simulink model "CDMA_RX_TX_with_UWA_pathloss_channel"  (Simulink 7.7)
settings: Solver=ode45  StartTime=0.0  StopTime=1  RelTol=1e-3
settings Model: Creator=iPRATEEK  LastModifiedBy=iPRATEEK

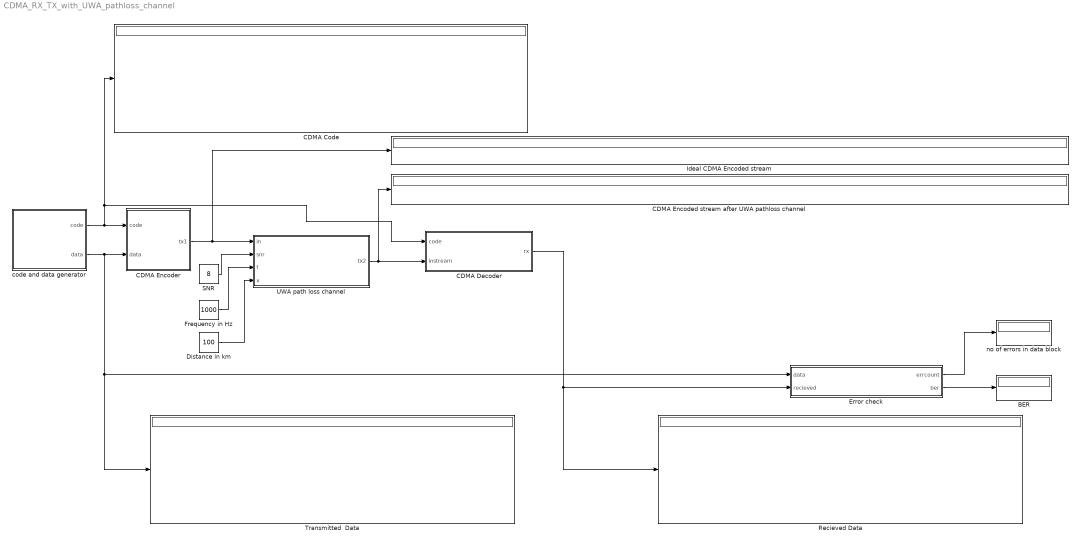
== system CDMA_RX_TX_with_UWA_pathloss_channel ==
  "BER " : Display
      settings: Format=short_e
  CDMA Code : Display
  CDMA Decoder : Stateflow chart  TreatAsAtomicUnit=on
  CDMA Encoded stream after UWA pathloss channel : Display
  CDMA Encoder : Stateflow chart  TreatAsAtomicUnit=on
  Distance in km : Constant  Value=100
  Error check : Stateflow chart  TreatAsAtomicUnit=on
  Frequency in Hz : Constant  Value=1000
  Ideal CDMA Encoded stream : Display
  Recieved Data : Display
  SNR : Constant  Value=8
  "Transmitted  Data " : Display
  UWA path loss channel : Stateflow chart  TreatAsAtomicUnit=on
  code and data generator : Stateflow chart  TreatAsAtomicUnit=on
  no of errors in data block : Display
  wires:
  code and data generator/1(code) -> CDMA Encoder/1(code), CDMA Decoder/1(code), CDMA Code/1
  code and data generator/2(data) -> CDMA Encoder/2(data), "Transmitted  Data "/1, Error check/1(data)
  CDMA Encoder/1(tx1) -> UWA path loss channel/1(in), Ideal CDMA Encoded stream/1
  SNR/1 -> UWA path loss channel/2(snr)
  CDMA Decoder/1(rx) -> Recieved Data/1, Error check/2(recieved)
  Error check/1(errcount) -> no of errors in data block/1
  Error check/2(ber) -> "BER "/1
  Frequency in Hz/1 -> UWA path loss channel/3(f)
  Distance in km/1 -> UWA path loss channel/4(x)
  UWA path loss channel/1(tx2) -> CDMA Decoder/2(instream), CDMA Encoded stream after UWA pathloss channel/1

== matlab function CDMA Encoder ==
  data: code input double; data input double size=[8,100]; tx1 output double
function tx1  = cdmaencoder(code,data)
data1=(data*2)-1;
y=zeros(8,800);
% [r,c]=size(data);
for i=1:8
y(i,:)=kron(data1(i,:),code(i,:));
end
tx1=sum(y);
end

== matlab function code and data generator ==
  data: code output double; data output double size=[8,100]
function [code,data] = codendatagen()
%#codegen
os=1;% increasing this value will improve ber

bits=100;
code=hadamard(8)
coder.extrinsic('randi')
data1=zeros(8,100)
data1=randi([0 1],8,100)
data=data1;

end

== matlab function UWA path loss channel ==
  data: in input double; tx2 output double; snr input double; f input double; x input double
function tx2 = uwapathlosschannel(in,snr,f,x)
tx=zeros(1,800)
coder.extrinsic('awgn');
tx=awgn(in,snr,'measured');
tx2=uwapathlosschannel(tx,f,x);
end


function[out]=uwapathlosschannel(in,f,x)
%%[out,gf,a,ax]=uwapathlosschannel(in)
%%out is data stream after path loss
%%ax is under water path loss 
%gf is the absorption coefficient
%f is freqeuncy it is assumed 1000hz 
%x is disatnce it is assumed 100km
%k is constant between 0.001 to 1
% f=input('');
k=.01;
% f=1000;
% x=100;
gf=(0.11*f^2/(1+f^2))+(44*f^2/(4100+f^2))+2.75*10^(-4)+0.003;%g(f)
a=exp(gf/10);
ax=x^k*a^x;%under water path loss 
out=in*ax;
end

== matlab function CDMA Decoder ==
  data: code input double; rx output double; instream input double
function rx =cdmadecoder(code,instream)
rx1=zeros(8,100);
for i=1:8
    x=kron(ones(1,100),code(i,:));
    x1=x.*instream;
    x2=reshape(x1,8,numel(x1)/8);
    x3=sum(x2);
    rx1(i,:)=x3;
end
rx=rx1>0;
end

== matlab function Error check ==
  data: data input double; errcount output double; recieved input double; ber output double
function[errcount,ber]=errorcount(data,recieved)
coder.extrinsic('biterr');
% a=zeros(800,1);
% b=zeros(800,1);
a=reshape(data,800,1);
b=reshape(recieved,800,1);
ber=zeros(1,1);
errcount=zeros(1,1);
[errcount,ber]=biterr(a,b);
end
